simulink model "MRAC_MIT_regulator"  (R2021b)
settings: Solver=VariableStepAuto  StartTime=0.0  StopTime=100  MaxStep=1e-2  RelTol=1e-3
undefined symbols (not defined in the file): alpha, am, bm, pGain, pT, upb
settings Model: Creator=miso  LastModifiedBy=Ondrej

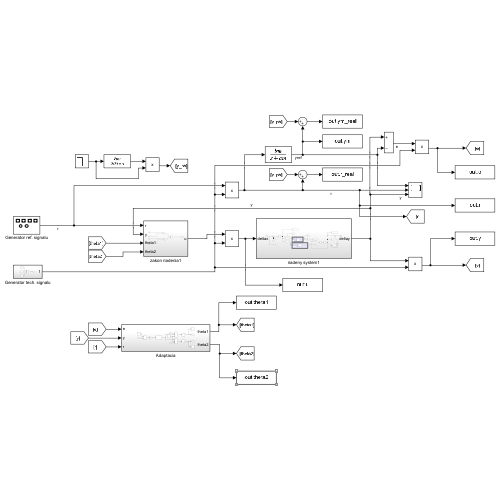
[thumbnail: Simulink's stored preview of the top-level diagram]
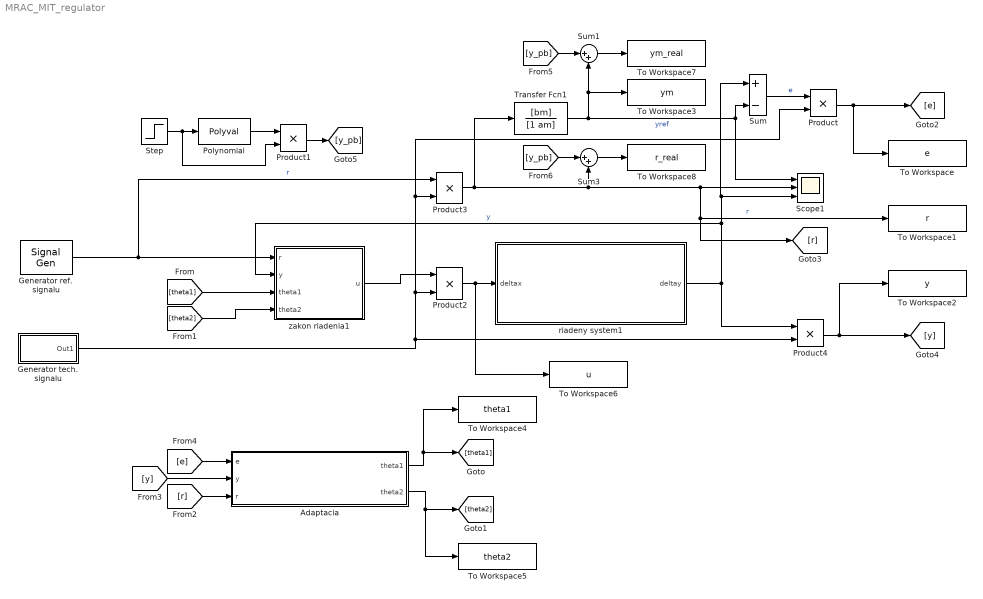
== system MRAC_MIT_regulator ==
  Adaptacia : Subsystem
  Generator ref. signalu : SignalGenerator  WaveForm=square  Amplitude=-6  Frequency=1/10
  Generator tech. signalu : Subsystem
  Polynomial : Polyval  Coefs=pGain
  Product{,1..4} (5 alike) : Product
  Scope1 : Scope  NumInputPorts=3
  Step : Step  Time=50  Before=upb  After=upb-upb_delta  SampleTime=0
  Sum : Sum  Inputs=+-
  Sum1 : Sum  Inputs=|++
  Sum3 : Sum  Inputs=|++
  To Workspace : ToWorkspace  VariableName=e  SaveFormat=Timeseries  SampleTime=-1
  To Workspace1 : ToWorkspace  VariableName=r  SaveFormat=Timeseries  SampleTime=-1
  To Workspace2 : ToWorkspace  VariableName=y  SaveFormat=Timeseries  SampleTime=-1
  To Workspace3 : ToWorkspace  VariableName=ym  SaveFormat=Timeseries  SampleTime=-1
  To Workspace4 : ToWorkspace  VariableName=theta1  SaveFormat=Timeseries  SampleTime=-1
  To Workspace5 : ToWorkspace  VariableName=theta2  SaveFormat=Timeseries  SampleTime=-1
  To Workspace6 : ToWorkspace  VariableName=u  SaveFormat=Timeseries  SampleTime=-1
  To Workspace7 : ToWorkspace  VariableName=ym_real  SaveFormat=Timeseries  SampleTime=-1
  To Workspace8 : ToWorkspace  VariableName=r_real  SaveFormat=Timeseries  SampleTime=-1
  Transfer Fcn1 : TransferFcn  Numerator=[bm]  Denominator=[1 am]
  riadeny system1 : Subsystem
  zakon riadenia1 : Subsystem
  wires:
  Product2/1 -> To Workspace6/1, riadeny system1/1(deltax)
  Transfer Fcn1/1 -> To Workspace3/1, Sum1/2, Scope1/1, Sum/2  "yref"
  Product3/1 -> Transfer Fcn1/1, Sum3/2, Scope1/2, [r], To Workspace1/1  "r"
  Generator ref. signalu/1 -> Product3/1, zakon riadenia1/1(r)  "r"
  zakon riadenia1/1(u) -> Product2/1
  riadeny system1/1(deltay) -> Product4/1, zakon riadenia1/2(y), Scope1/3, Sum/1  "y"
  [theta1] -> zakon riadenia1/3(theta1)
  [theta2] -> zakon riadenia1/4(theta2)
  Product4/1 -> [y], To Workspace2/1
  Sum/1 -> Product/1  "e"
  Product/1 -> To Workspace/1, [e]
  Step/1 -> Product1/2, Polynomial/1
  [y_pb] -> Sum1/1
  Sum1/1 -> To Workspace7/1
  Sum3/1 -> To Workspace8/1
  [y_pb] -> Sum3/1
  Polynomial/1 -> Product1/1
  Product1/1 -> [y_pb]
  [e] -> Adaptacia/1(e)
  [y] -> Adaptacia/2(y)
  [r] -> Adaptacia/3(r)
  Adaptacia/2(theta2) -> [theta2], To Workspace5/1
  Adaptacia/1(theta1) -> [theta1], To Workspace4/1
  Generator tech. signalu/1(Out1) -> Product4/2, Product2/2, Product/2, Product3/2

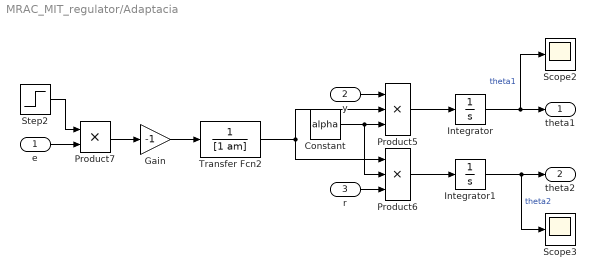
== system MRAC_MIT_regulator/Adaptacia ==
  e : Inport
  y : Inport  Port=2
  r : Inport  Port=3
  Constant : Constant  Value=alpha
  Gain : Gain  Gain=-1
  Integrator : Integrator
  Integrator1 : Integrator
  Product5 : Product  Inputs=3
  Product6 : Product  Inputs=3
  Product7 : Product
  Scope2 : Scope
  Scope3 : Scope
  Step2 : Step  Time=100  Before=1  After=0  SampleTime=0
  Transfer Fcn2 : TransferFcn  Denominator=[1 am]
  theta1 : Outport
  theta2 : Outport  Port=2
  wires:
  Gain/1 -> Transfer Fcn2/1
  Integrator/1 -> theta1/1, Scope2/1  "theta1"
  Integrator1/1 -> theta2/1, Scope3/1  "theta2"
  Constant/1 -> Product6/2, Product5/3
  Product5/1 -> Integrator/1
  y/1 -> Product5/1
  r/1 -> Product6/3
  Transfer Fcn2/1 -> Product5/2, Product6/1
  Product7/1 -> Gain/1
  Product6/1 -> Integrator1/1
  Step2/1 -> Product7/1
  e/1 -> Product7/2

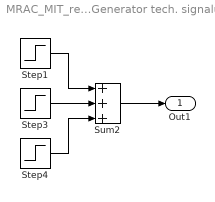
== system MRAC_MIT_regulator/Generator tech. signalu ==
  Step1 : Step  Time=10  SampleTime=0
  Step3 : Step  Time=45  Before=1  After=0  SampleTime=0
  Step4 : Step  Time=60  Before=-1  After=0  SampleTime=0
  Sum2 : Sum  Inputs=+++
  Out1 : Outport
  wires:
  Step3/1 -> Sum2/2
  Step4/1 -> Sum2/3
  Step1/1 -> Sum2/1
  Sum2/1 -> Out1/1

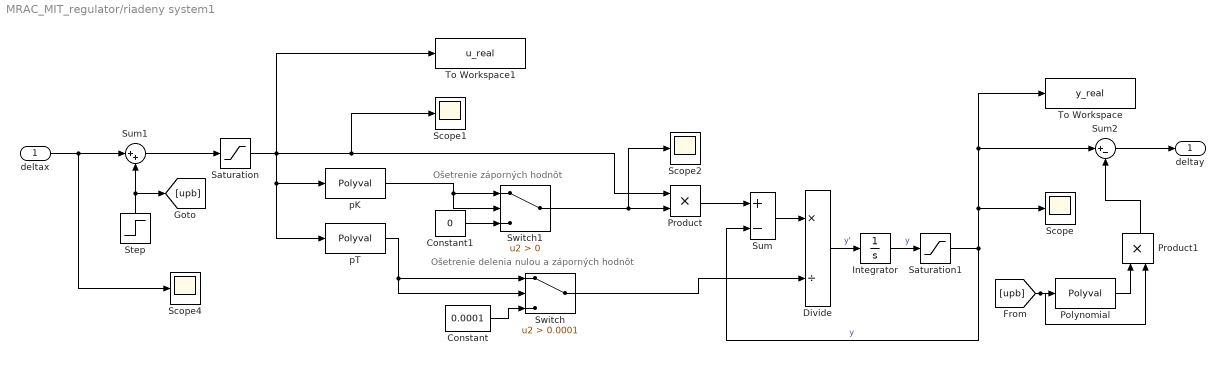
== system MRAC_MIT_regulator/riadeny system1 ==
  note: Ošetrenie delenia nulou a záporných hodnôt
  note: Ošetrenie záporných hodnôt
  deltax : Inport
  Constant : Constant  Value=0.0001
  Constant1 : Constant  Value=0
  Divide : Product  Inputs=*/
  Integrator : Integrator
  Polynomial : Polyval  Coefs=pGain
  Product : Product
  Product1 : Product
  Saturation : Saturate  UpperLimit=255  LowerLimit=0
  Saturation1 : Saturate  UpperLimit=1023  LowerLimit=0
  Scope{,1..2,4} (4 alike) : Scope
  Step : Step  Time=50  Before=upb  After=upb-upb_delta  SampleTime=0
  Sum : Sum  Inputs=+-
  Sum1 : Sum  Inputs=|++
  Sum2 : Sum  Inputs=|+-
  Switch : Switch  Criteria=u2 > Threshold  Threshold=0.0001
  Switch1 : Switch  Criteria=u2 > Threshold
  To Workspace : ToWorkspace  VariableName=y_real  SaveFormat=Timeseries  SampleTime=-1
  To Workspace1 : ToWorkspace  VariableName=u_real  SaveFormat=Timeseries  SampleTime=-1
  pK : Polyval  Coefs=pGain
  pT : Polyval  Coefs=pT
  deltay : Outport
  wires:
  Sum/1 -> Divide/1
  Saturation1/1 -> To Workspace/1, Sum2/1, Scope/1, Sum/2  "y"
  Constant/1 -> Switch/3
  pT/1 -> Switch/1, Switch/2
  pK/1 -> Switch1/2, Switch1/1
  Switch/1 -> Divide/2
  Constant1/1 -> Switch1/3
  Product/1 -> Sum/1
  Switch1/1 -> Scope2/1, Product/2
  Integrator/1 -> Saturation1/1  "y"
  Divide/1 -> Integrator/1  "y'"
  deltax/1 -> Scope4/1, Sum1/1
  Sum1/1 -> Saturation/1
  Saturation/1 -> To Workspace1/1, pT/1, pK/1, Scope1/1, Product/1
  Sum2/1 -> deltay/1
  Polynomial/1 -> Product1/1
  Step/1 -> [upb], Sum1/2
  [upb] -> Product1/2, Polynomial/1
  Product1/1 -> Sum2/2

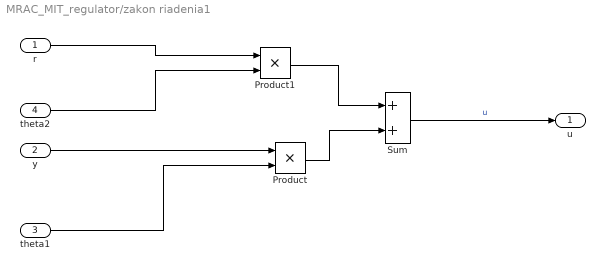
== system MRAC_MIT_regulator/zakon riadenia1 ==
  r : Inport
  y : Inport  Port=2
  theta1 : Inport  Port=3
  theta2 : Inport  Port=4
  Product : Product
  Product1 : Product
  Sum : Sum
  u : Outport
  wires:
  Product1/1 -> Sum/1
  Product/1 -> Sum/2
  y/1 -> Product/1
  Sum/1 -> u/1  "u"
  r/1 -> Product1/1
  theta1/1 -> Product/2
  theta2/1 -> Product1/2
